simulink model "SF049A_LoaMgr"  (R2013b)
settings: Solver=FixedStepDiscrete  SolverMode=SingleTasking  StartTime=0.0  StopTime=1  FixedStep=0.002  RelTol=1e-3
undefined symbols (not defined in the file): CURRMEASLOAMTGTNMASK_CNT_U08, IVTRLOAMTGTNMASK_CNT_U08, LoaCtrldShtdwn, LoaCurrMeasIdptSigNrFlt, LoaHwTqIdptSigNrFlt, LoaImdtShtdwn, LoaIvtrIdptSigNrFlt, LOAMAXSLEW_ULSPERSEC_F32, LoaMgrCurrIvtrMtgtnRate, LoaMgrCurrIvtrMtgtnSca, LoaMgrCurrIvtrMtgtnScaZeroEna, LoaMgrCurrMeasIdptSig0Resp, LoaMgrCurrMeasIdptSig1Resp, LoaMgrCurrMeasIdptSig2Resp, LoaMgrCurrMeasIdptSigFltThd, LoaMgrCurrMeasMtgtnRate, LoaMgrCurrMeasMtgtnSca, LoaMgrCurrMeasMtgtnScaZeroEna, LoaMgrFadeOutStRate, LoaMgrHwTqIdptSig0NoTqLoaResp, LoaMgrHwTqIdptSig1NoTqLoaResp, LoaMgrHwTqIdptSig2Resp, LoaMgrHwTqIdptSig4Resp, LoaMgrHwTqIdptSigFltThd, LoaMgrHwTqLoaAvlResp, LoaMgrIvtrIdptSig0Resp, LoaMgrIvtrIdptSig1Resp, LoaMgrIvtrIdptSig2Resp, LoaMgrIvtrIdptSigFltThd, LoaMgrIvtrMtgtnRate, LoaMgrIvtrMtgtnSca, LoaMgrIvtrMtgtnScaZeroEna, LoaMgrLimdStRate, LoaMgrLimdStSca, LoaMgrMotAgAvlSnsrlsResp, LoaMgrMotAgIdptSig0NoSnsrlsResp, LoaMgrMotAgIdptSig1NoSnsrlsResp, LoaMgrMotAgIdptSig2Resp, LoaMgrMotAgIdptSig3Resp, LoaMgrMotAgIdptSigFltThd, LoaMgrMotAgMtgtnRate, LoaMgrMotAgMtgtnSca, LoaMgrMotAgMtgtnScaZeroEna, LoaMotAgIdptSigNrFlt, LOASCAONE_ULS_F32, LOASCAZERO_ULS_F32, LoaSt1, LOASTIMDTSHTDWN_CNT_U08, LOASTNORM_CNT_U08, LOASTSWMTGTN_CNT_U08, MAXCURRMEASIDPTSIGALLWD_CNT_U08, MAXHWTQIDPTSIGALLWD_CNT_U08, MAXIVTRIDPTSIGALLWD_CNT_U08, MAXMOTAGMECLIDPTSIGALLWD_CNT_U08, NODEBSTEP_CNT_U16, NtcSts1, SigQlfr1
libraries: simulink x30, NxtrMin x4, NxtrMax x4, NxtrLim x2
(part 1 of 7)
settings Model: Creator=TZ5743  LastModifiedBy=BZHF94
settings SolverCC: AutoInsertRateTranBlk=on  InsertRTBMode=Always
settings DataIOCC: LimitDataPoints=off  SaveFormat=Structure  ReturnWorkspaceOutputs=on
settings OptimizationCC: BlockReduction=off  DefaultParameterBehavior=Inlined  ZeroExternalMemoryAtStartup=off  ZeroInternalMemoryAtStartup=off  OptimizeModelRefInitCode=on  LifeSpan=1  SimCompilerOptimization=off
settings DebuggingCC: SignalInfNanChecking=error  SignalRangeChecking=warning  UnderspecifiedInitializationDetection=Simplified  MergeDetectMultiDrivingBlocksExec=error  SolverPrmCheckMsg=error  InheritedTsInSrcMsg=error  SingleTaskRateTransMsg=error  TasksWithSamePriorityMsg=error  SigSpecEnsureSampleTimeMsg=error  CheckMatrixSingularityMsg=error  ParameterUnderflowMsg=error  ParameterPrecisionLossMsg=error  ParameterTunabilityLossMsg=error  FixptConstUnderflowMsg=warning  FixptConstOverflowMsg=warning  VectorMatrixConversionMsg=error  SignalLabelMismatchMsg=error  UnconnectedInputMsg=error  UnconnectedOutputMsg=error  UnconnectedLineMsg=error  SFcnCompatibilityMsg=error  FrameProcessingCompatibilityMsg=error  UniqueDataStoreMsg=warning  BusObjectLabelMismatch=error  RootOutportRequireBusObject=error  AssertControl=DisableAll  AllowSymbolicDim=off  ModelReferenceIOMsg=error  ModelReferenceVersionMismatchMessage=warning  ModelReferenceIOMismatchMessage=error  ModelReferenceDataLoggingMessage=error  StateNameClashWarn=warning  StrictBusMsg=ErrorOnBusTreatedAsVector  NonBusSignalsTreatedAsBus=error  SFUnexpectedBacktrackingDiag=error  SFInvalidInputDataAccessInChartInitDiag=error  SFNoUnconditionalDefaultTransitionDiag=error  SFTransitionOutsideNaturalParentDiag=error  SFUnconditionalTransitionShadowingDiag=error  SFUndirectedBroadcastEventsDiag=error
settings ModelReferenceCC: ModelReferenceNumInstancesAllowed=Single
settings RTWCC: SystemTargetFile=autosar.tlc  GenCodeOnly=on  TemplateMakefile=ert_default_tmf  Description=AUTOSAR  GenerateReport=on  LaunchReport=on  RTWCompilerOptimization=off
settings CodeAppCC: GenerateComments=off  IgnoreCustomStorageClasses=off  CustomSymbolStrType=$N$R$M  CustomSymbolStrBlkIO=$N$M  SimulinkBlockComments=off
settings STFCustomTargetCC: CodeReplacementLibrary=None  ParMdlRefBuildCompliant=on  CompOptLevelCompliant=on  IncludeMdlTerminateFcn=off  CombineOutputUpdateFcns=on  SuppressErrorStatus=on  ERTFirstTimeCompliant=on  ERTCustomFileBanners=on  SupportNonFinite=off  SupportComplex=off  SupportContinuousTime=off  SupportNonInlinedSFcns=off  MATLABClassNameForMDSCustomization=Simulink.SoftwareTarget.ERTCustomization  AutosarCompliant=on  GRTInterface=off  UseToolchainInfoCompliant=on  SystemTargetFile=autosar.tlc
settings ERTTargetCC: ConcurrentExecutionCompliant=off  IncludeMdlTerminateFcn=off  SuppressErrorStatus=on  SupportNonFinite=off  SupportComplex=off  ModelStepFunctionPrototypeControlCompliant=off  CPPClassGenCompliant=off  AutosarCompliant=on  InlinedParameterPlacement=NonHierarchical  ERTCustomFileTemplate=example_file_process.tlc  EnableUserReplacementTypes=on
settings ConfigComp: CovMetricSettings=dw  CovHtmlReporting=on  CovSaveCumulativeToWorkspaceVar=on  CovSaveSingleToWorkspaceVar=on  CovModelRefEnable=Off  CovExternalEMLEnable=off

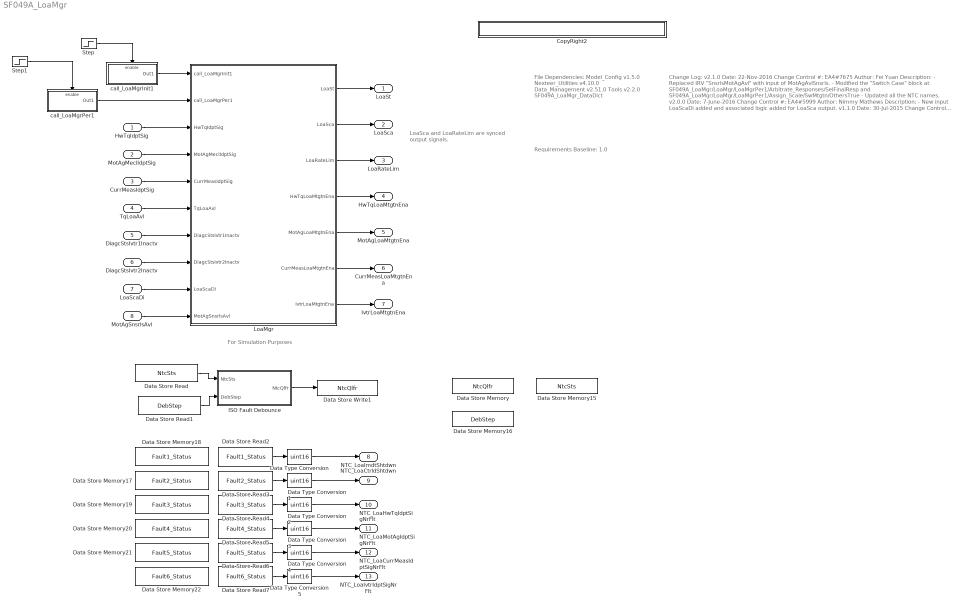
== system SF049A_LoaMgr ==
  note: LoaSca and LoaRateLim are synced
      | output signals.
  note: File Dependencies:
      |
      | Model_Config v1.5.0
      | Nexteer_Utilities v4.10.0
      | Data_Management v2.51.0
      | Tools v2.2.0
      | SF049A_LoaMgr_DataDict
  note: Requirements Baseline: 1.0
  note: Change Log:
      |
      | v2.1.0
      | Date: 22-Nov-2016
      | Change Control #: EA4#7675
      | Author: Fei Yuan
      | Description:
      | - Replaced IRV "SnsrlsMotAgAvl" with input of MotAgAvlSnsrls.
      | - Modified the "Switch Case" block at
      | SF049A_LoaMgr/LoaMgr/LoaMgrPer1/Arbitrate_Responses/SelFinalResp and
      | SF049A_LoaMgr/LoaMgr/LoaMgrPer1/Assign_Scale/SwMtgtn/OthersTrue
      | - Updated all the NTC names.
      |
      | v2.0.0
      | Date: 7-June-2016
      | Change Control #: 	EA4#5999
      | Author:  Nimmy Mathews
      | Description:
      | - New input LoaScaDi added and associated logic added for
      | LoaSca output.
      |
      | v1.1.0
      | Date: 30-Jul-2015
      | Change Control #: EA4#947
      | DRW:  Sudeep Shankar
      | Description:
      | - Initial Release based off of EA3 Version v1.1.0
      | - Output Signal name correction
  note: For Simulation Purposes
  HwTqIdptSig : Inport  RequirementInfo={} %GIDa_c0ada7cc_2a84_41fc_944b_6b17ef65ea9c
  MotAgMeclIdptSig : Inport  RequirementInfo={} %GIDa_73372f4d_c568_47db_aad1_8b4638be1747  Port=2
  CurrMeasIdptSig : Inport  RequirementInfo={} %GIDa_84af9224_d287_43ff_b284_7e5ed6dfb324  Port=3
  TqLoaAvl : Inport  RequirementInfo={} %GIDa_93076217_93fd_4cef_a21d_6480a5a63a27  Port=4
  DiagcStsIvtr1Inactv : Inport  RequirementInfo={} %GIDa_3739eb85_24f0_476e_b882_4900d0ef3f73  Port=5
  DiagcStsIvtr2Inactv : Inport  RequirementInfo={} %GIDa_5f578b66_4982_413b_90dc_34bab3afd1d1  Port=6
  LoaScaDi : Inport  RequirementInfo={} %GIDa_13ee9f09_c993_4f8a_825d_b1ce3d1d2719  Port=7
  MotAgSnsrlsAvl : Inport  RequirementInfo={} %GIDa_1b4fe355_7a68_40b3_bc8e_ac797fbd4766  Port=8
  CopyRight2 : Subsystem  Description=|  mask(Copyright Information){none=on}
      | Copyright info block.                                               
      |                                                                     
      | Place copyright information at the top of every subsystem in design.
      mask prompts: none "No parameters"
      mask help: Place copyright information at the top of every subsystem in design.
      mask Display:
      | NxtrConf = 'Nexteer Confidential';
      | 
      | sys = bdroot; %handle for the current model ("system")
      | first = get_param(sys,'Created');
      | if(isempty(first))
      |     first = datestr(now,'yyyy');
      | else
      |     first = first(end-3:end);  %year is last four digits
      | end
      | 
      | last = get_param(sys,'LastModifiedDate');
      | if isempty(last)
      |     last = datestr(now,'yyyy');
      | else
      |     last = last(end-3:end);
      | end
      | 
      | if strcmp(first,last)
      |     fprintf('%s -- Copyright %s Nexteer',NxtrConf,first)
      | else
      |     fprintf('%s -- %s%s- %s Nexteer',NxtrConf,char(169),first,last)
      | end
  Data Store Memory : DataStoreMemory  DataStoreName=NtcQlfr  OutDataTypeStr=uint8
  Data Store Memory15 : DataStoreMemory  DataStoreName=NtcSts  InitialValue=NtcSts1.NTCSTS_PREPASSD
  Data Store Memory16 : DataStoreMemory  DataStoreName=DebStep
  Data Store Memory17 : DataStoreMemory  DataStoreName=Fault2_Status  InitialValue=NtcSts1.NTCSTS_PASSD  OutDataTypeStr=Enum: NtcSts1
  Data Store Memory18 : DataStoreMemory  DataStoreName=Fault1_Status  InitialValue=NtcSts1.NTCSTS_PASSD  OutDataTypeStr=Enum: NtcSts1
  Data Store Memory19 : DataStoreMemory  DataStoreName=Fault3_Status  InitialValue=NtcSts1.NTCSTS_PASSD  OutDataTypeStr=Enum: NtcSts1
  Data Store Memory20 : DataStoreMemory  DataStoreName=Fault4_Status  InitialValue=NtcSts1.NTCSTS_PASSD  OutDataTypeStr=Enum: NtcSts1
  Data Store Memory21 : DataStoreMemory  DataStoreName=Fault5_Status  InitialValue=NtcSts1.NTCSTS_PASSD  OutDataTypeStr=Enum: NtcSts1
  Data Store Memory22 : DataStoreMemory  DataStoreName=Fault6_Status  InitialValue=NtcSts1.NTCSTS_PASSD  OutDataTypeStr=Enum: NtcSts1
  Data Store Read : DataStoreRead  DataStoreName=NtcSts  SampleTime=0.004
  Data Store Read1 : DataStoreRead  DataStoreName=DebStep  SampleTime=0.004
  Data Store Read2 : DataStoreRead  DataStoreName=Fault1_Status  SampleTime=.004
  Data Store Read3 : DataStoreRead  DataStoreName=Fault2_Status  SampleTime=.004
  Data Store Read4 : DataStoreRead  DataStoreName=Fault3_Status  SampleTime=.004
  Data Store Read5 : DataStoreRead  DataStoreName=Fault4_Status  SampleTime=.004
  Data Store Read6 : DataStoreRead  DataStoreName=Fault5_Status  SampleTime=.004
  Data Store Read7 : DataStoreRead  DataStoreName=Fault6_Status  SampleTime=0.004
  Data Store Write1 : DataStoreWrite  DataStoreName=NtcQlfr
  Data Type Conversion{,1..5} (6 alike) : DataTypeConversion  OutDataTypeStr=uint16
  ISO Fault Debounce : Subsystem  mask(SetNTC){}
      mask help: For Simulation Purposes
  LoaMgr : Subsystem
  Step : Step  Time=.0001  Before=1  After=0  SampleTime=0
  Step1 : Step  Time=.004  SampleTime=0
  call_LoaMgrInit1 : Subsystem  TreatAsAtomicUnit=on
  call_LoaMgrPer1 : Subsystem  TreatAsAtomicUnit=on
  LoaSt : Outport  RequirementInfo={} %GIDa_93bae52a_8cb1_4bd9_a2c4_d588b7d059cf
  LoaSca : Outport  RequirementInfo={} %GIDa_8c460775_12f6_4528_9f51_57ca189e85fc  Port=2
  LoaRateLim : Outport  RequirementInfo={} %GIDa_ffab9872_1ea4_4ffd_9e16_324c719cb008  Port=3
  HwTqLoaMtgtnEna : Outport  RequirementInfo={} %GIDa_b272817b_3ff3_4259_b745_ea4cd35b806a  Port=4
  MotAgLoaMtgtnEna : Outport  RequirementInfo={} %GIDa_98224876_72c1_4d11_a238_725dcb00f091  Port=5
  CurrMeasLoaMtgtnEna : Outport  RequirementInfo={} %GIDa_771c3727_c0e3_4c42_9260_a180eb374e5c  Port=6
  IvtrLoaMtgtnEna : Outport  RequirementInfo={} %GIDa_ccb9de9c_ade8_4e48_bfad_57a91e3cbf19  Port=7
  NTC_LoaImdtShtdwn : Outport  Port=8
  NTC_LoaCtrldShtdwn : Outport  Port=9
  NTC_LoaHwTqIdptSigNrFlt : Outport  Port=10
  NTC_LoaMotAgIdptSigNrFlt : Outport  Port=11
  NTC_LoaCurrMeasIdptSigNrFlt : Outport  Port=12
  NTC_LoaIvtrIdptSigNrFlt : Outport  Port=13
  wires:
  HwTqIdptSig/1 -> LoaMgr/3(HwTqIdptSig)
  MotAgMeclIdptSig/1 -> LoaMgr/4(MotAgMeclIdptSig)
  CurrMeasIdptSig/1 -> LoaMgr/5(CurrMeasIdptSig)
  DiagcStsIvtr1Inactv/1 -> LoaMgr/7(DiagcStsIvtr1Inactv)
  TqLoaAvl/1 -> LoaMgr/6(TqLoaAvl)
  DiagcStsIvtr2Inactv/1 -> LoaMgr/8(DiagcStsIvtr2Inactv)
  LoaMgr/7(IvtrLoaMtgtnEna) -> IvtrLoaMtgtnEna/1
  LoaMgr/6(CurrMeasLoaMtgtnEna) -> CurrMeasLoaMtgtnEna/1
  LoaMgr/5(MotAgLoaMtgtnEna) -> MotAgLoaMtgtnEna/1
  LoaMgr/4(HwTqLoaMtgtnEna) -> HwTqLoaMtgtnEna/1
  LoaMgr/3(LoaRateLim) -> LoaRateLim/1
  LoaMgr/2(LoaSca) -> LoaSca/1
  LoaMgr/1(LoaSt) -> LoaSt/1
  call_LoaMgrInit1/1(Out1) -> LoaMgr/1(call_LoaMgrInit1)
  Step/1 -> call_LoaMgrInit1/Enable
  Data Store Read2/1 -> Data Type Conversion/1
  Data Type Conversion/1 -> NTC_LoaImdtShtdwn/1
  Data Store Read3/1 -> Data Type Conversion1/1
  Data Type Conversion1/1 -> NTC_LoaCtrldShtdwn/1
  Data Store Read4/1 -> Data Type Conversion2/1
  Data Type Conversion2/1 -> NTC_LoaHwTqIdptSigNrFlt/1
  Data Type Conversion3/1 -> NTC_LoaMotAgIdptSigNrFlt/1
  Data Type Conversion4/1 -> NTC_LoaCurrMeasIdptSigNrFlt/1
  Data Store Read5/1 -> Data Type Conversion3/1
  Data Store Read6/1 -> Data Type Conversion4/1
  Data Type Conversion5/1 -> NTC_LoaIvtrIdptSigNrFlt/1
  Data Store Read7/1 -> Data Type Conversion5/1
  ISO Fault Debounce/1(NtcQlfr) -> Data Store Write1/1
  Data Store Read/1 -> ISO Fault Debounce/1(NtcSts)
  Data Store Read1/1 -> ISO Fault Debounce/2(DebStep)
  LoaScaDi/1 -> LoaMgr/9(LoaScaDi)
  MotAgSnsrlsAvl/1 -> LoaMgr/10(MotAgSnsrlsAvl)
  Step1/1 -> call_LoaMgrPer1/Enable
  call_LoaMgrPer1/1(Out1) -> LoaMgr/2(call_LoaMgrPer1)

== system SF049A_LoaMgr/CopyRight2 ==

== system SF049A_LoaMgr/ISO Fault Debounce ==
  note: Note:
      |
      | - "ISO Fault Debounce Design" Simulink block intent to use here for Simulation purpose only. Do not Code this block
  NtcSts : Inport
  DebStep : Inport  Port=2
  Constant : Constant  Value=false
  CopyRight2 : Subsystem  Description=|  mask(Copyright Information){none=on}
      | Copyright info block.                                               
      |                                                                     
      | Place copyright information at the top of every subsystem in design.
      mask prompts: none "No parameters"
      mask help: Place copyright information at the top of every subsystem in design.
      mask Display:
      | NxtrConf = 'Nexteer Confidential';
      | 
      | sys = bdroot; %handle for the current model ("system")
      | first = get_param(sys,'Created');
      | first = first(end-3:end);  %year is last four digits
      | 
      | last = get_param(sys,'LastModifiedDate');
      | if isempty(last)
      |     last = datestr(now,'yyyy');
      | else
      |     last = last(end-3:end);
      | end
      | 
      | if strcmp(first,last)
      |     fprintf('%s -- Copyright %s Nexteer',NxtrConf,first)
      | else
      |     fprintf('%s -- %s%s- %s Nexteer',NxtrConf,char(169),first,last)
      | end
  Data Type Conversion : DataTypeConversion
  DiagMgr : Subsystem  RequirementInfo={} %GIDa_61294fe9_bc00_4ee8_bc9f_a9abb89fc5dc
  Ground : Ground
  Terminator : Terminator
  NtcQlfr : Outport
  wires:
  Ground/1 -> DiagMgr/3(SvcClr)
  DebStep/1 -> DiagMgr/2(DebStep)
  NtcSts/1 -> DiagMgr/1(NtcSts)
  Constant/1 -> DiagMgr/4(Recoverable)
  Data Type Conversion/1 -> NtcQlfr/1
  DiagMgr/1(Qualifier) -> Data Type Conversion/1
  DiagMgr/2(ErrAcc) -> Terminator/1

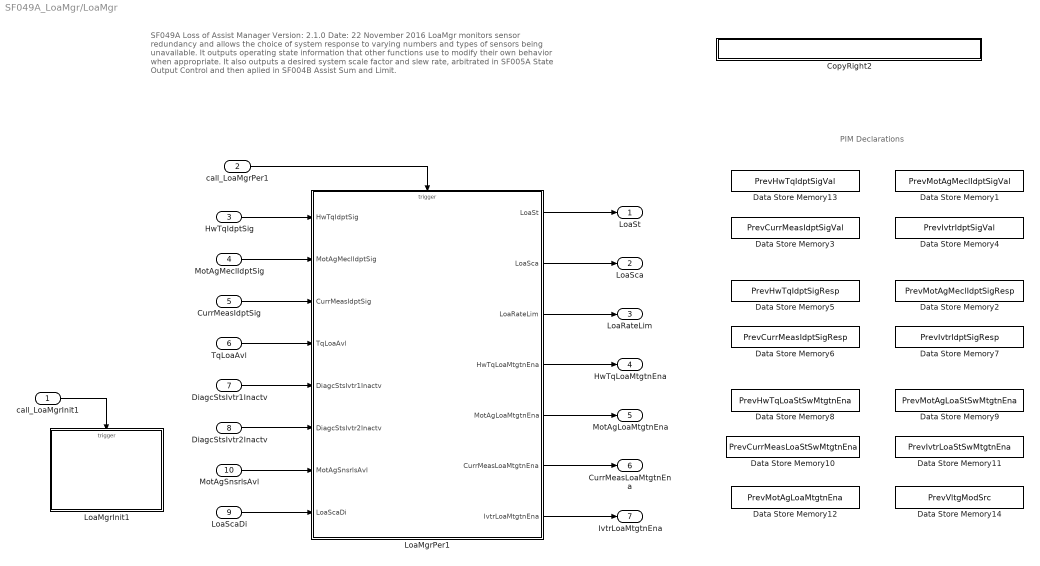
== system SF049A_LoaMgr/LoaMgr ==
  note: SF049A  Loss of Assist Manager       Version: 2.1.0                                                       Date:  22 November 2016
      |
      | LoaMgr monitors sensor redundancy and allows the choice of system response to varying numbers and types of sensors being unavailable.  It
      | outputs operating state information that other functions use to modify their own behavior when appropriate.  It also outputs a desired system
      | scale factor and slew rate, arbitrated in SF005A State Output Control and then aplied in SF004B Assist Sum and Limit.
  note: PIM Declarations
  call_LoaMgrInit1 : Inport
  call_LoaMgrPer1 : Inport  RequirementInfo="{'linktype_rmi_doors' '00012fd5 (/E-STEER Core/SubSystem Specifications/Application Functions - EA4/SF049A Loss of Assist Manager)' '#SF049A_161' 'true' 'REQ:  SF049A_161' '' } %GIDa_11a999fa_4307_4876_8422_1fdf0f90e9d7"  Port=2
  HwTqIdptSig : Inport  RequirementInfo="{'linktype_rmi_doors' '00012fd5 (/E-STEER Core/SubSystem Specifications/Application Functions - EA4/SF049A Loss of Assist Manager)' '#SF049A_9' 'true' 'REQ:  SF049A_9' '' } %GIDa_e136a68a_be9b_41e2_8d19_731d1b546a22"  Port=3
  MotAgMeclIdptSig : Inport  RequirementInfo="{'linktype_rmi_doors' '00012fd5 (/E-STEER Core/SubSystem Specifications/Application Functions - EA4/SF049A Loss of Assist Manager)' '#SF049A_10' 'true' 'REQ:  SF049A_10' '' } %GIDa_03485ada_2d02_4097_843d_27b3dd3d89ce"  Port=4
  CurrMeasIdptSig : Inport  RequirementInfo="{'linktype_rmi_doors' '00012fd5 (/E-STEER Core/SubSystem Specifications/Application Functions - EA4/SF049A Loss of Assist Manager)' '#SF049A_11' 'true' 'REQ:  SF049A_11' '' } %GIDa_b13fb45e_c676_4df0_b1a7_3991e4929c24"  Port=5
  TqLoaAvl : Inport  RequirementInfo="{'linktype_rmi_doors' '00012fd5 (/E-STEER Core/SubSystem Specifications/Application Functions - EA4/SF049A Loss of Assist Manager)' '#SF049A_12' 'true' 'REQ:  SF049A_12' '' } %GIDa_ad428560_d84e_4090_8b2c_395c8b1d79f4"  Port=6
  DiagcStsIvtr1Inactv : Inport  RequirementInfo="{'linktype_rmi_doors' '00012fd5 (/E-STEER Core/SubSystem Specifications/Application Functions - EA4/SF049A Loss of Assist Manager)' '#SF049A_13' 'true' 'REQ:  SF049A_13' '' } %GIDa_a09d3721_2ae3_425a_97fe_a373142e0df8"  Port=7
  DiagcStsIvtr2Inactv : Inport  RequirementInfo="{'linktype_rmi_doors' '00012fd5 (/E-STEER Core/SubSystem Specifications/Application Functions - EA4/SF049A Loss of Assist Manager)' '#SF049A_14' 'true' 'REQ:  SF049A_14' '' } %GIDa_37cf1e87_9470_44c4_ae46_3d3e796de4ab"  Port=8
  LoaScaDi : Inport  RequirementInfo="{'linktype_rmi_doors' '00012fd5 (/E-STEER Core/SubSystem Specifications/Application Functions - EA4/SF049A Loss of Assist Manager)' '#SF049A_15' 'true' 'REQ:  SF049A_15' '' } %GIDa_542c339e_a191_413c_b7b4_dd829497f318"  Port=9
  MotAgSnsrlsAvl : Inport  RequirementInfo="{'linktype_rmi_doors' '00012fd5 (/E-STEER Core/SubSystem Specifications/Application Functions - EA4/SF049A Loss of Assist Manager)' '#SF049A_164' 'true' 'REQ:  SF049A_164' '' } %GIDa_fe7b95aa_5b28_4b7e_a407_a916842b11d1"  Port=10
  CopyRight2 : Subsystem  Description=|  mask(Copyright Information){none=on}
      | Copyright info block.                                               
      |                                                                     
      | Place copyright information at the top of every subsystem in design.
      mask prompts: none "No parameters"
      mask help: Place copyright information at the top of every subsystem in design.
      mask Display:
      | NxtrConf = 'Nexteer Confidential';
      | 
      | sys = bdroot; %handle for the current model ("system")
      | first = get_param(sys,'Created');
      | first = first(end-3:end);  %year is last four digits
      | 
      | last = get_param(sys,'LastModifiedDate');
      | if isempty(last)
      |     last = datestr(now,'yyyy');
      | else
      |     last = last(end-3:end);
      | end
      | 
      | if strcmp(first,last)
      |     fprintf('%s -- Copyright %s Nexteer',NxtrConf,first)
      | else
      |     fprintf('%s -- %s%s- %s Nexteer',NxtrConf,char(169),first,last)
      | end
  Data Store Memory1 : DataStoreMemory  DataStoreName=PrevMotAgMeclIdptSigVal  StateMustResolveToSignalObject=on
  Data Store Memory10 : DataStoreMemory  DataStoreName=PrevCurrMeasLoaStSwMtgtnEna  StateMustResolveToSignalObject=on
  Data Store Memory11 : DataStoreMemory  DataStoreName=PrevIvtrLoaStSwMtgtnEna  StateMustResolveToSignalObject=on
  Data Store Memory12 : DataStoreMemory  DataStoreName=PrevMotAgLoaMtgtnEna  StateMustResolveToSignalObject=on
  Data Store Memory13 : DataStoreMemory  DataStoreName=PrevHwTqIdptSigVal  StateMustResolveToSignalObject=on
  Data Store Memory14 : DataStoreMemory  DataStoreName=PrevVltgModSrc  StateMustResolveToSignalObject=on
  Data Store Memory2 : DataStoreMemory  DataStoreName=PrevMotAgMeclIdptSigResp  StateMustResolveToSignalObject=on
  Data Store Memory3 : DataStoreMemory  DataStoreName=PrevCurrMeasIdptSigVal  StateMustResolveToSignalObject=on
  Data Store Memory4 : DataStoreMemory  DataStoreName=PrevIvtrIdptSigVal  StateMustResolveToSignalObject=on
  Data Store Memory5 : DataStoreMemory  DataStoreName=PrevHwTqIdptSigResp  StateMustResolveToSignalObject=on
  Data Store Memory6 : DataStoreMemory  DataStoreName=PrevCurrMeasIdptSigResp  StateMustResolveToSignalObject=on
  Data Store Memory7 : DataStoreMemory  DataStoreName=PrevIvtrIdptSigResp  StateMustResolveToSignalObject=on
  Data Store Memory8 : DataStoreMemory  DataStoreName=PrevHwTqLoaStSwMtgtnEna  StateMustResolveToSignalObject=on
  Data Store Memory9 : DataStoreMemory  DataStoreName=PrevMotAgLoaStSwMtgtnEna  StateMustResolveToSignalObject=on
  LoaMgrInit1 : Subsystem  TreatAsAtomicUnit=on
  LoaMgrPer1 : Subsystem
  LoaSt : Outport  RequirementInfo="{'linktype_rmi_doors' '00012fd5 (/E-STEER Core/SubSystem Specifications/Application Functions - EA4/SF049A Loss of Assist Manager)' '#SF049A_17' 'true' 'REQ:  SF049A_17' '' } %GIDa_485d87b4_d02d_47fa_b823_48b3336f7452"
  LoaSca : Outport  RequirementInfo="{'linktype_rmi_doors' '00012fd5 (/E-STEER Core/SubSystem Specifications/Application Functions - EA4/SF049A Loss of Assist Manager)' '#SF049A_18' 'true' 'REQ:  SF049A_18' '' } %GIDa_0bd5c46e_7ba7_4668_acb6_e4652e0a23fd"  Port=2
  LoaRateLim : Outport  RequirementInfo="{'linktype_rmi_doors' '00012fd5 (/E-STEER Core/SubSystem Specifications/Application Functions - EA4/SF049A Loss of Assist Manager)' '#SF049A_19' 'true' 'REQ:  SF049A_19' '' } %GIDa_80797401_dd21_4a69_8582_3227909dc8d3"  Port=3
  HwTqLoaMtgtnEna : Outport  RequirementInfo="{'linktype_rmi_doors' '00012fd5 (/E-STEER Core/SubSystem Specifications/Application Functions - EA4/SF049A Loss of Assist Manager)' '#SF049A_20' 'true' 'REQ:  SF049A_20' '' } %GIDa_f23d32ba_f930_49ed_92e7_19e481e9c810"  Port=4
  MotAgLoaMtgtnEna : Outport  RequirementInfo="{'linktype_rmi_doors' '00012fd5 (/E-STEER Core/SubSystem Specifications/Application Functions - EA4/SF049A Loss of Assist Manager)' '#SF049A_21' 'true' 'REQ:  SF049A_21' '' } %GIDa_58615b08_5037_4791_88b8_f139534e2d3d"  Port=5
  CurrMeasLoaMtgtnEna : Outport  RequirementInfo="{'linktype_rmi_doors' '00012fd5 (/E-STEER Core/SubSystem Specifications/Application Functions - EA4/SF049A Loss of Assist Manager)' '#SF049A_22' 'true' 'REQ:  SF049A_22' '' } %GIDa_49e649da_286c_497e_8c32_683faa7a42a6"  Port=6
  IvtrLoaMtgtnEna : Outport  RequirementInfo="{'linktype_rmi_doors' '00012fd5 (/E-STEER Core/SubSystem Specifications/Application Functions - EA4/SF049A Loss of Assist Manager)' '#SF049A_23' 'true' 'REQ:  SF049A_23' '' } %GIDa_de65f1b1_1a81_47b6_87b6_d026873f8ac5"  Port=7
  wires:
  LoaScaDi/1 -> LoaMgrPer1/8(LoaScaDi)
  LoaMgrPer1/1(LoaSt) -> LoaSt/1
  LoaMgrPer1/2(LoaSca) -> LoaSca/1
  LoaMgrPer1/3(LoaRateLim) -> LoaRateLim/1
  LoaMgrPer1/4(HwTqLoaMtgtnEna) -> HwTqLoaMtgtnEna/1
  LoaMgrPer1/5(MotAgLoaMtgtnEna) -> MotAgLoaMtgtnEna/1
  LoaMgrPer1/6(CurrMeasLoaMtgtnEna) -> CurrMeasLoaMtgtnEna/1
  LoaMgrPer1/7(IvtrLoaMtgtnEna) -> IvtrLoaMtgtnEna/1
  call_LoaMgrPer1/1 -> LoaMgrPer1/Trigger
  MotAgMeclIdptSig/1 -> LoaMgrPer1/2(MotAgMeclIdptSig)
  HwTqIdptSig/1 -> LoaMgrPer1/1(HwTqIdptSig)
  TqLoaAvl/1 -> LoaMgrPer1/4(TqLoaAvl)
  DiagcStsIvtr1Inactv/1 -> LoaMgrPer1/5(DiagcStsIvtr1Inactv)
  CurrMeasIdptSig/1 -> LoaMgrPer1/3(CurrMeasIdptSig)
  DiagcStsIvtr2Inactv/1 -> LoaMgrPer1/6(DiagcStsIvtr2Inactv)
  call_LoaMgrInit1/1 -> LoaMgrInit1/Trigger
  MotAgSnsrlsAvl/1 -> LoaMgrPer1/7(MotAgSnsrlsAvl)

== system SF049A_LoaMgr/call_LoaMgrInit1 ==
  Enable : EnablePort
  CopyRight2 : Subsystem  Description=|  mask(Copyright Information){none=on}
      | Copyright info block.                                               
      |                                                                     
      | Place copyright information at the top of every subsystem in design.
      mask prompts: none "No parameters"
      mask help: Place copyright information at the top of every subsystem in design.
      mask Display:
      | NxtrConf = 'Nexteer Confidential';
      | 
      | sys = bdroot; %handle for the current model ("system")
      | first = get_param(sys,'Created');
      | if(isempty(first))
      |     first = datestr(now,'yyyy');
      | else
      |     first = first(end-3:end);  %year is last four digits
      | end
      | 
      | last = get_param(sys,'LastModifiedDate');
      | if isempty(last)
      |     last = datestr(now,'yyyy');
      | else
      |     last = last(end-3:end);
      | end
      | 
      | if strcmp(first,last)
      |     fprintf('%s -- Copyright %s Nexteer',NxtrConf,first)
      | else
      |     fprintf('%s -- %s%s- %s Nexteer',NxtrConf,char(169),first,last)
      | end
  Function-Call Generator : simulink/Ports & Subsystems/Function-Call Generator  sample_time=0  numberOfIterations=1
  Out1 : Outport
  wires:
  Function-Call Generator/1 -> Out1/1

== system SF049A_LoaMgr/call_LoaMgrPer1 ==
  Enable : EnablePort
  CopyRight2 : Subsystem  Description=|  mask(Copyright Information){none=on}
      | Copyright info block.                                               
      |                                                                     
      | Place copyright information at the top of every subsystem in design.
      mask prompts: none "No parameters"
      mask help: Place copyright information at the top of every subsystem in design.
      mask Display:
      | NxtrConf = 'Nexteer Confidential';
      | 
      | sys = bdroot; %handle for the current model ("system")
      | first = get_param(sys,'Created');
      | if(isempty(first))
      |     first = datestr(now,'yyyy');
      | else
      |     first = first(end-3:end);  %year is last four digits
      | end
      | 
      | last = get_param(sys,'LastModifiedDate');
      | if isempty(last)
      |     last = datestr(now,'yyyy');
      | else
      |     last = last(end-3:end);
      | end
      | 
      | if strcmp(first,last)
      |     fprintf('%s -- Copyright %s Nexteer',NxtrConf,first)
      | else
      |     fprintf('%s -- %s%s- %s Nexteer',NxtrConf,char(169),first,last)
      | end
  Function-Call Generator : simulink/Ports & Subsystems/Function-Call Generator  sample_time=0.004  numberOfIterations=1
  Out1 : Outport
  wires:
  Function-Call Generator/1 -> Out1/1

== system SF049A_LoaMgr/ISO Fault Debounce/CopyRight2 ==

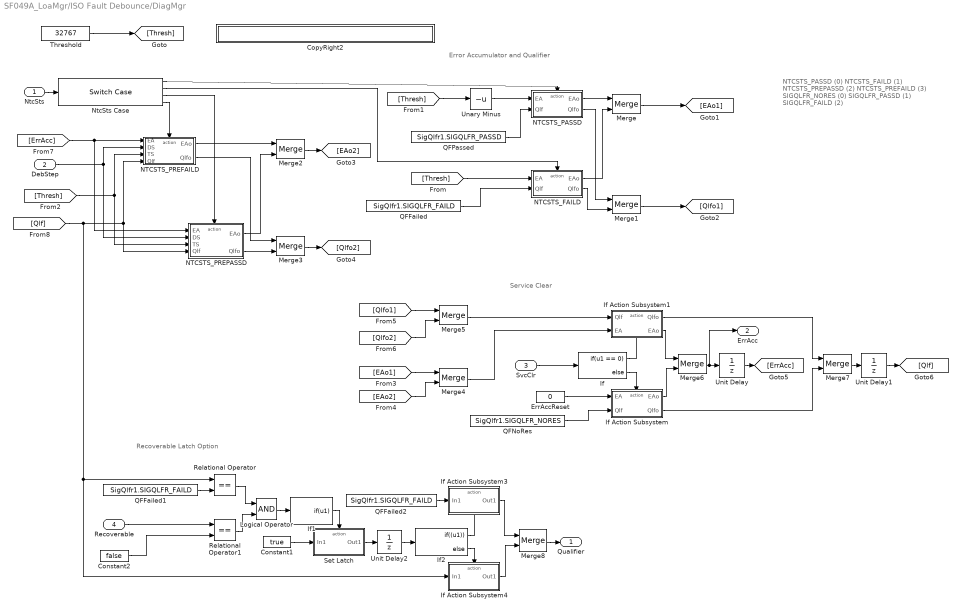
== system SF049A_LoaMgr/ISO Fault Debounce/DiagMgr ==
  note: NTCSTS_PASSD         (0)
      | NTCSTS_FAILD           (1)
      | NTCSTS_PREPASSD  (2)
      | NTCSTS_PREFAILD    (3)
      |
      | SIGQLFR_NORES       (0)
      | SIGQLFR_PASSD        (1)
      | SIGQLFR_FAILD          (2)
  note: Error Accumulator and Qualifier
  note: Service Clear
  note: Recoverable Latch Option
  NtcSts : Inport
  DebStep : Inport  Port=2
  SvcClr : Inport  Port=3
  Recoverable : Inport  Port=4
  Constant1 : Constant  Value=true  OutDataTypeStr=boolean
  Constant2 : Constant  Value=false  OutDataTypeStr=boolean
  CopyRight2 : Subsystem  Description=|  mask(Copyright Information){none=on}
      | Copyright info block.                                               
      |                                                                     
      | Place copyright information at the top of every subsystem in design.
      mask prompts: none "No parameters"
      mask help: Place copyright information at the top of every subsystem in design.
      mask Display:
      | NxtrConf = 'Nexteer Confidential';
      | 
      | sys = bdroot; %handle for the current model ("system")
      | first = get_param(sys,'Created');
      | first = first(end-3:end);  %year is last four digits
      | 
      | last = get_param(sys,'LastModifiedDate');
      | if isempty(last)
      |     last = datestr(now,'yyyy');
      | else
      |     last = last(end-3:end);
      | end
      | 
      | if strcmp(first,last)
      |     fprintf('%s -- Copyright %s Nexteer',NxtrConf,first)
      | else
      |     fprintf('%s -- %s%s- %s Nexteer',NxtrConf,char(169),first,last)
      | end
  ErrAccReset : Constant  Value=0
  If : If  IfExpression=u1 == 0
  If Action Subsystem : Subsystem  TreatAsAtomicUnit=on
  If Action Subsystem1 : Subsystem  TreatAsAtomicUnit=on
  If Action Subsystem3 : Subsystem  TreatAsAtomicUnit=on
  If Action Subsystem4 : Subsystem  TreatAsAtomicUnit=on
  If1 : If  IfExpression=u1  ShowElse=off
  If2 : If  IfExpression=(u1)
  Logical Operator : Logic  AllPortsSameDT=off  OutDataTypeStr=boolean
  Merge{,1..8} (9 alike) : Merge
  NTCSTS_FAILD : Subsystem  TreatAsAtomicUnit=on
  NTCSTS_PASSD : Subsystem  TreatAsAtomicUnit=on
  NTCSTS_PREFAILD : Subsystem  TreatAsAtomicUnit=on
  NTCSTS_PREPASSD : Subsystem  TreatAsAtomicUnit=on
  NtcSts Case : SwitchCase  CaseConditions={NtcSts1.NTCSTS_PASSD,NtcSts1.NTCSTS_FAILD,NtcSts1.NTCSTS_PREPASSD,NtcSts1.NTCSTS_PREFAILD}  ShowDefaultCase=off
  QFFailed : Constant  Value=SigQlfr1.SIGQLFR_FAILD  OutDataTypeStr=Enum: SigQlfr1
  QFFailed1 : Constant  Value=SigQlfr1.SIGQLFR_FAILD  OutDataTypeStr=Enum: SigQlfr1
  QFFailed2 : Constant  Value=SigQlfr1.SIGQLFR_FAILD  OutDataTypeStr=Enum: SigQlfr1
  QFNoRes : Constant  Value=SigQlfr1.SIGQLFR_NORES  OutDataTypeStr=Enum: SigQlfr1
  QFPassed : Constant  Value=SigQlfr1.SIGQLFR_PASSD  OutDataTypeStr=Enum: SigQlfr1
  Relational Operator : RelationalOperator  Operator===  OutDataTypeStr=boolean
      settings: AttributesFormatString=Qualifier Failed
  Relational Operator1 : RelationalOperator  Operator===  OutDataTypeStr=boolean
      settings: AttributesFormatString=Recoverable False
  Set Latch : Subsystem  TreatAsAtomicUnit=on
  Threshold : Constant  Value=32767
  Unary Minus : UnaryMinus
  Unit Delay : UnitDelay  SampleTime=-1
  Unit Delay1 : UnitDelay  InitialCondition=SigQlfr1.SIGQLFR_NORES  SampleTime=-1  StateName=SigQlfr1
  Unit Delay2 : UnitDelay  SampleTime=-1
  Qualifier : Outport
  ErrAcc : Outport  Port=2
  wires:
  DebStep/1 -> NTCSTS_PREPASSD/2(DS), NTCSTS_PREFAILD/2(DS)
  NtcSts Case/3 -> NTCSTS_PREPASSD/Action
  If/2 -> If Action Subsystem/Action
  QFPassed/1 -> NTCSTS_PASSD/2(Qlf)
  If2/1 -> If Action Subsystem3/Action
  If2/2 -> If Action Subsystem4/Action
  [Thresh] -> NTCSTS_FAILD/1(EA)
  QFFailed/1 -> NTCSTS_FAILD/2(Qlf)
  If Action Subsystem4/1(Out1) -> Merge8/2
  Merge8/1 -> Qualifier/1
  QFFailed2/1 -> If Action Subsystem3/1(In1)
  Unit Delay2/1 -> If2/1
  NtcSts Case/1 -> NTCSTS_PASSD/Action
  NtcSts Case/4 -> NTCSTS_PREFAILD/Action
  SvcClr/1 -> If/1
  NtcSts Case/2 -> NTCSTS_FAILD/Action
  [Thresh] -> Unary Minus/1
  [Thresh] -> NTCSTS_PREPASSD/3(TS), NTCSTS_PREFAILD/3(TS)
  NTCSTS_PREFAILD/2(Qlfo) -> Merge3/1
  [ErrAcc] -> NTCSTS_PREPASSD/1(EA), NTCSTS_PREFAILD/1(EA)
  NTCSTS_PREPASSD/1(EAo) -> Merge2/2
  NTCSTS_FAILD/1(EAo) -> Merge/2
  NTCSTS_FAILD/2(Qlfo) -> Merge1/2
  If Action Subsystem3/1(Out1) -> Merge8/1
  [Qlfo1] -> Merge5/1
  NTCSTS_PREPASSD/2(Qlfo) -> Merge3/2
  NTCSTS_PREFAILD/1(EAo) -> Merge2/1
  [Qlfo2] -> Merge5/2
  [EAo1] -> Merge4/1
  [Qlf] -> Relational Operator/1, If Action Subsystem4/1(In1), NTCSTS_PREFAILD/4(Qlf), NTCSTS_PREPASSD/4(Qlf)
  [EAo2] -> Merge4/2
  Merge/1 -> [EAo1]
  ErrAccReset/1 -> If Action Subsystem/1(EA)
  QFNoRes/1 -> If Action Subsystem/2(Qlf)
  Merge6/1 -> ErrAcc/1, Unit Delay/1
  If Action Subsystem1/2(EAo) -> Merge6/1
  Merge4/1 -> If Action Subsystem1/2(EA)
  If/1 -> If Action Subsystem1/Action
  If Action Subsystem1/1(Qlfo) -> Merge7/1
  NTCSTS_PASSD/2(Qlfo) -> Merge1/1
  Threshold/1 -> [Thresh]
  If Action Subsystem/1(EAo) -> Merge6/2
  NTCSTS_PASSD/1(EAo) -> Merge/1
  If Action Subsystem/2(Qlfo) -> Merge7/2
  Merge1/1 -> [Qlfo1]
  Merge2/1 -> [EAo2]
  Merge3/1 -> [Qlfo2]
  Merge5/1 -> If Action Subsystem1/1(Qlf)
  NtcSts/1 -> NtcSts Case/1
  Unit Delay/1 -> [ErrAcc]
  Unit Delay1/1 -> [Qlf]
  Merge7/1 -> Unit Delay1/1
  Relational Operator/1 -> Logical Operator/1
  Relational Operator1/1 -> Logical Operator/2
  Constant2/1 -> Relational Operator1/2
  Logical Operator/1 -> If1/1
  If1/1 -> Set Latch/Action
  Constant1/1 -> Set Latch/1(In1)
  QFFailed1/1 -> Relational Operator/2
  Set Latch/1(Out1) -> Unit Delay2/1
  Recoverable/1 -> Relational Operator1/1
  Unary Minus/1 -> NTCSTS_PASSD/1(EA)

== system SF049A_LoaMgr/LoaMgr/CopyRight2 ==

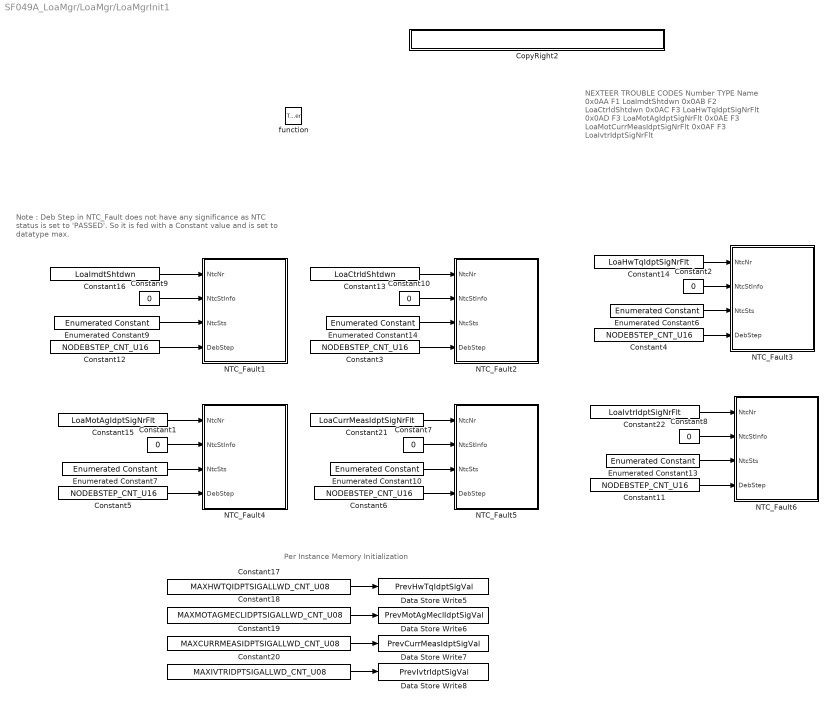
== system SF049A_LoaMgr/LoaMgr/LoaMgrInit1 ==
  note: Per Instance Memory Initialization
  note: NEXTEER TROUBLE CODES
      | Number  TYPE   Name
      |  0x0AA      F1      LoaImdtShtdwn
      |  0x0AB      F2      LoaCtrldShtdwn
      |  0x0AC      F3      LoaHwTqIdptSigNrFlt
      |  0x0AD      F3      LoaMotAgIdptSigNrFlt
      |  0x0AE      F3      LoaMotCurrMeasIdptSigNrFlt
      |  0x0AF      F3      LoaIvtrIdptSigNrFlt
  note: Note : Deb Step in NTC_Fault does not have any significance as
      | NTC status is set to 'PASSED'. So it is fed with a Constant value and
      | is set to datatype max.
  function : TriggerPort  TriggerType=function-call
  Constant1 : Constant  RequirementInfo="{'linktype_rmi_doors' '00012fd5 (/E-STEER Core/SubSystem Specifications/Application Functions - EA4/SF049A Loss of Assist Manager)' '#SF049A_68' 'true' 'REQ:  SF049A_68' '' } %GIDa_09a72554_6b8b_4627_b610_7c880b96c152"  Value=0
  Constant10 : Constant  RequirementInfo="{'linktype_rmi_doors' '00012fd5 (/E-STEER Core/SubSystem Specifications/Application Functions - EA4/SF049A Loss of Assist Manager)' '#SF049A_46' 'true' 'REQ:  SF049A_46' '' } %GIDa_2780d869_b7d4_4c52_8148_a5ebd8a8c128"  Value=0
  Constant11 : Constant  RequirementInfo="{'linktype_rmi_doors' '00012fd5 (/E-STEER Core/SubSystem Specifications/Application Functions - EA4/SF049A Loss of Assist Manager)' '#SF049A_90' 'true' 'REQ:  SF049A_90' '' } %GIDa_8760c850_a166_4f26_aeef_3d69371a50e7"  Value=NODEBSTEP_CNT_U16
  Constant12 : Constant  RequirementInfo="{'linktype_rmi_doors' '00012fd5 (/E-STEER Core/SubSystem Specifications/Application Functions - EA4/SF049A Loss of Assist Manager)' '#SF049A_35' 'true' 'REQ:  SF049A_35' '' } %GIDa_d176be49_c6f2_4e13_b18e_1b05a48376bf"  Value=NODEBSTEP_CNT_U16
  Constant13 : Constant  RequirementInfo="{'linktype_rmi_doors' '00012fd5 (/E-STEER Core/SubSystem Specifications/Application Functions - EA4/SF049A Loss of Assist Manager)' '#SF049A_46' 'true' 'REQ:  SF049A_46' '' } %GIDa_6c547535_063b_445c_af94_eb5574f08747"  Value=LoaCtrldShtdwn
  Constant14 : Constant  RequirementInfo="{'linktype_rmi_doors' '00012fd5 (/E-STEER Core/SubSystem Specifications/Application Functions - EA4/SF049A Loss of Assist Manager)' '#SF049A_57' 'true' 'REQ:  SF049A_57' '' } %GIDa_6c0d8de0_c077_4a89_b170_495f4d0daf45"  Value=LoaHwTqIdptSigNrFlt
  Constant15 : Constant  RequirementInfo="{'linktype_rmi_doors' '00012fd5 (/E-STEER Core/SubSystem Specifications/Application Functions - EA4/SF049A Loss of Assist Manager)' '#SF049A_68' 'true' 'REQ:  SF049A_68' '' } %GIDa_f4e97660_4a45_4ee8_aefd_216a590e907f"  Value=LoaMotAgIdptSigNrFlt
  Constant16 : Constant  RequirementInfo="{'linktype_rmi_doors' '00012fd5 (/E-STEER Core/SubSystem Specifications/Application Functions - EA4/SF049A Loss of Assist Manager)' '#SF049A_35' 'true' 'REQ:  SF049A_35' '' } %GIDa_ee2f095f_e9fa_486e_ae86_a30232b53fb4"  Value=LoaImdtShtdwn
  Constant17 : Constant  RequirementInfo={} %GIDa_5b950255_8f18_4912_81dd_eb91606197df  Value=MAXHWTQIDPTSIGALLWD_CNT_U08  OutDataTypeStr=uint8
  Constant18 : Constant  RequirementInfo={} %GIDa_54c005ab_4540_429a_9970_f23d45e39613  Value=MAXMOTAGMECLIDPTSIGALLWD_CNT_U08  OutDataTypeStr=uint8
  Constant19 : Constant  RequirementInfo={} %GIDa_947a6b5f_12de_441e_bcec_6b3f89217e6d  Value=MAXCURRMEASIDPTSIGALLWD_CNT_U08  OutDataTypeStr=uint8
  Constant2 : Constant  RequirementInfo="{'linktype_rmi_doors' '00012fd5 (/E-STEER Core/SubSystem Specifications/Application Functions - EA4/SF049A Loss of Assist Manager)' '#SF049A_57' 'true' 'REQ:  SF049A_57' '' } %GIDa_83264d8f_e7cf_4e36_a77c_cbe9ece48f33"  Value=0
  Constant20 : Constant  RequirementInfo={} %GIDa_07837d8e_9d24_42c2_b79b_cfda2d14c87d  Value=MAXIVTRIDPTSIGALLWD_CNT_U08  OutDataTypeStr=uint8
  Constant21 : Constant  RequirementInfo="{'linktype_rmi_doors' '00012fd5 (/E-STEER Core/SubSystem Specifications/Application Functions - EA4/SF049A Loss of Assist Manager)' '#SF049A_79' 'true' 'REQ:  SF049A_79' '' } %GIDa_0ddbf860_f1d0_48af_9661_f573615d1661"  Value=LoaCurrMeasIdptSigNrFlt
  Constant22 : Constant  RequirementInfo="{'linktype_rmi_doors' '00012fd5 (/E-STEER Core/SubSystem Specifications/Application Functions - EA4/SF049A Loss of Assist Manager)' '#SF049A_90' 'true' 'REQ:  SF049A_90' '' } %GIDa_9c0928f8_bb13_48cc_a72b_c39958c4c501"  Value=LoaIvtrIdptSigNrFlt
  Constant3 : Constant  RequirementInfo="{'linktype_rmi_doors' '00012fd5 (/E-STEER Core/SubSystem Specifications/Application Functions - EA4/SF049A Loss of Assist Manager)' '#SF049A_46' 'true' 'REQ:  SF049A_46' '' } %GIDa_0bf69534_0956_44cc_9c2a_433bc6c27e43"  Value=NODEBSTEP_CNT_U16
  Constant4 : Constant  RequirementInfo="{'linktype_rmi_doors' '00012fd5 (/E-STEER Core/SubSystem Specifications/Application Functions - EA4/SF049A Loss of Assist Manager)' '#SF049A_57' 'true' 'REQ:  SF049A_57' '' } %GIDa_0fa24ea6_9c16_40ba_9b81_9df4de3ddc47"  Value=NODEBSTEP_CNT_U16
  Constant5 : Constant  RequirementInfo="{'linktype_rmi_doors' '00012fd5 (/E-STEER Core/SubSystem Specifications/Application Functions - EA4/SF049A Loss of Assist Manager)' '#SF049A_68' 'true' 'REQ:  SF049A_68' '' } %GIDa_29c9f302_3383_4bbb_86ad_bd7246db1c6a"  Value=NODEBSTEP_CNT_U16
  Constant6 : Constant  RequirementInfo="{'linktype_rmi_doors' '00012fd5 (/E-STEER Core/SubSystem Specifications/Application Functions - EA4/SF049A Loss of Assist Manager)' '#SF049A_79' 'true' 'REQ:  SF049A_79' '' } %GIDa_693eee1d_940e_4510_b6ca_b2e09a33882e"  Value=NODEBSTEP_CNT_U16
  Constant7 : Constant  RequirementInfo="{'linktype_rmi_doors' '00012fd5 (/E-STEER Core/SubSystem Specifications/Application Functions - EA4/SF049A Loss of Assist Manager)' '#SF049A_79' 'true' 'REQ:  SF049A_79' '' } %GIDa_bd597d58_e2c2_4d46_a831_7ad8a2d0c9f8"  Value=0
  Constant8 : Constant  RequirementInfo="{'linktype_rmi_doors' '00012fd5 (/E-STEER Core/SubSystem Specifications/Application Functions - EA4/SF049A Loss of Assist Manager)' '#SF049A_90' 'true' 'REQ:  SF049A_90' '' } %GIDa_66b775bc_b9d9_40ba_b454_434fd06622b7"  Value=0
  Constant9 : Constant  RequirementInfo="{'linktype_rmi_doors' '00012fd5 (/E-STEER Core/SubSystem Specifications/Application Functions - EA4/SF049A Loss of Assist Manager)' '#SF049A_35' 'true' 'REQ:  SF049A_35' '' } %GIDa_7a457627_e162_4cd9_b6f0_06929f77b0ee"  Value=0
  CopyRight2 : Subsystem  Description=|  mask(Copyright Information){none=on}
      | Copyright info block.                                               
      |                                                                     
      | Place copyright information at the top of every subsystem in design.
      mask prompts: none "No parameters"
      mask help: Place copyright information at the top of every subsystem in design.
      mask Display:
      | NxtrConf = 'Nexteer Confidential';
      | 
      | sys = bdroot; %handle for the current model ("system")
      | first = get_param(sys,'Created');
      | first = first(end-3:end);  %year is last four digits
      | 
      | last = get_param(sys,'LastModifiedDate');
      | if isempty(last)
      |     last = datestr(now,'yyyy');
      | else
      |     last = last(end-3:end);
      | end
      | 
      | if strcmp(first,last)
      |     fprintf('%s -- Copyright %s Nexteer',NxtrConf,first)
      | else
      |     fprintf('%s -- %s%s- %s Nexteer',NxtrConf,char(169),first,last)
      | end
  Data Store Write5 : DataStoreWrite  RequirementInfo={} %GIDa_6608b05c_0683_4793_b206_c046e47d2e17  DataStoreName=PrevHwTqIdptSigVal
  Data Store Write6 : DataStoreWrite  RequirementInfo={} %GIDa_7f471370_469d_423d_8316_5f647dac324c  DataStoreName=PrevMotAgMeclIdptSigVal
  Data Store Write7 : DataStoreWrite  RequirementInfo={} %GIDa_ff2dc782_9d50_4d1d_a106_f1a00891ebf8  DataStoreName=PrevCurrMeasIdptSigVal
  Data Store Write8 : DataStoreWrite  RequirementInfo={} %GIDa_82eaf6ef_b4dd_4627_9b7c_307f23025eff  DataStoreName=PrevIvtrIdptSigVal
  Enumerated Constant10 : simulink/Sources/Enumerated Constant  RequirementInfo="{'linktype_rmi_doors' '00012fd5 (/E-STEER Core/SubSystem Specifications/Application Functions - EA4/SF049A Loss of Assist Manager)' '#SF049A_79' 'true' 'REQ:  SF049A_79' '' } %GIDa_b526159a_7605_418a_8f6c_df09f8ab0f2e"  OutDataTypeStr=Enum: NtcSts1  Value=NtcSts1.NTCSTS_PASSD  SampleTime=inf
  Enumerated Constant13 : simulink/Sources/Enumerated Constant  RequirementInfo="{'linktype_rmi_doors' '00012fd5 (/E-STEER Core/SubSystem Specifications/Application Functions - EA4/SF049A Loss of Assist Manager)' '#SF049A_90' 'true' 'REQ:  SF049A_90' '' } %GIDa_d3e6efb1_efb4_427f_b5b5_516029acb430"  OutDataTypeStr=Enum: NtcSts1  Value=NtcSts1.NTCSTS_PASSD  SampleTime=inf
  Enumerated Constant14 : simulink/Sources/Enumerated Constant  RequirementInfo="{'linktype_rmi_doors' '00012fd5 (/E-STEER Core/SubSystem Specifications/Application Functions - EA4/SF049A Loss of Assist Manager)' '#SF049A_46' 'true' 'REQ:  SF049A_46' '' } %GIDa_c0c65592_9d54_46fb_86ce_f75ee339a4f0"  OutDataTypeStr=Enum: NtcSts1  Value=NtcSts1.NTCSTS_PASSD  SampleTime=inf
  Enumerated Constant6 : simulink/Sources/Enumerated Constant  RequirementInfo="{'linktype_rmi_doors' '00012fd5 (/E-STEER Core/SubSystem Specifications/Application Functions - EA4/SF049A Loss of Assist Manager)' '#SF049A_57' 'true' 'REQ:  SF049A_57' '' } %GIDa_35a763d2_042b_4007_a721_954fca523208"  OutDataTypeStr=Enum: NtcSts1  Value=NtcSts1.NTCSTS_PASSD  SampleTime=inf
  Enumerated Constant7 : simulink/Sources/Enumerated Constant  RequirementInfo="{'linktype_rmi_doors' '00012fd5 (/E-STEER Core/SubSystem Specifications/Application Functions - EA4/SF049A Loss of Assist Manager)' '#SF049A_68' 'true' 'REQ:  SF049A_68' '' } %GIDa_351ce1e7_b97b_403a_a411_28e1e89dcaf0"  OutDataTypeStr=Enum: NtcSts1  Value=NtcSts1.NTCSTS_PASSD  SampleTime=inf
  Enumerated Constant9 : simulink/Sources/Enumerated Constant  RequirementInfo="{'linktype_rmi_doors' '00012fd5 (/E-STEER Core/SubSystem Specifications/Application Functions - EA4/SF049A Loss of Assist Manager)' '#SF049A_35' 'true' 'REQ:  SF049A_35' '' } %GIDa_30de0318_7c37_4833_8d7b_7440b72a791d"  OutDataTypeStr=Enum: NtcSts1  Value=NtcSts1.NTCSTS_PASSD  SampleTime=inf
  NTC_Fault1 : Subsystem  RequirementInfo="{'linktype_rmi_doors' '00012fd5 (/E-STEER Core/SubSystem Specifications/Application Functions - EA4/SF049A Loss of Assist Manager)' '#SF049A_35' 'true' 'REQ:  SF049A_35' '' } %GIDa_a11aadfb_dddf_46de_834c_f65b067005f1"  mask(SetNTC){}
      mask help: SetNTC library block
  NTC_Fault2 : Subsystem  RequirementInfo="{'linktype_rmi_doors' '00012fd5 (/E-STEER Core/SubSystem Specifications/Application Functions - EA4/SF049A Loss of Assist Manager)' '#SF049A_46' 'true' 'REQ:  SF049A_46' '' } %GIDa_297ee9a4_b750_4631_af05_5b9d8d57969c"  mask(SetNTC){}
      mask help: SetNTC library block
  NTC_Fault3 : Subsystem  RequirementInfo="{'linktype_rmi_doors' '00012fd5 (/E-STEER Core/SubSystem Specifications/Application Functions - EA4/SF049A Loss of Assist Manager)' '#SF049A_57' 'true' 'REQ:  SF049A_57' '' } %GIDa_1a5739c7_318f_4ab5_8a5c_73d329586bde"  mask(SetNTC){}
      mask help: SetNTC library block
  NTC_Fault4 : Subsystem  RequirementInfo="{'linktype_rmi_doors' '00012fd5 (/E-STEER Core/SubSystem Specifications/Application Functions - EA4/SF049A Loss of Assist Manager)' '#SF049A_68' 'true' 'REQ:  SF049A_68' '' } %GIDa_1b246348_21bd_45ae_852b_8bbdfb8cae08"  mask(SetNTC){}
      mask help: SetNTC library block
  NTC_Fault5 : Subsystem  RequirementInfo="{'linktype_rmi_doors' '00012fd5 (/E-STEER Core/SubSystem Specifications/Application Functions - EA4/SF049A Loss of Assist Manager)' '#SF049A_79' 'true' 'REQ:  SF049A_79' '' } %GIDa_796fa8cf_8bbd_45c3_b0fb_56c3c4bb3441"  mask(SetNTC){}
      mask help: SetNTC library block
  NTC_Fault6 : Subsystem  RequirementInfo="{'linktype_rmi_doors' '00012fd5 (/E-STEER Core/SubSystem Specifications/Application Functions - EA4/SF049A Loss of Assist Manager)' '#SF049A_90' 'true' 'REQ:  SF049A_90' '' } %GIDa_a3e32d5c_31c5_476e_951c_0fe301f50025"  mask(SetNTC){}
      mask help: SetNTC library block
  wires:
  Constant3/1 -> NTC_Fault2/4(DebStep)
  Enumerated Constant14/1 -> NTC_Fault2/3(NtcSts)
  Constant13/1 -> NTC_Fault2/1(NtcNr)
  Constant10/1 -> NTC_Fault2/2(NtcStInfo)
  Constant12/1 -> NTC_Fault1/4(DebStep)
  Enumerated Constant9/1 -> NTC_Fault1/3(NtcSts)
  Constant9/1 -> NTC_Fault1/2(NtcStInfo)
  Constant16/1 -> NTC_Fault1/1(NtcNr)
  Constant11/1 -> NTC_Fault6/4(DebStep)
  Enumerated Constant13/1 -> NTC_Fault6/3(NtcSts)
  Constant8/1 -> NTC_Fault6/2(NtcStInfo)
  Constant22/1 -> NTC_Fault6/1(NtcNr)
  Constant6/1 -> NTC_Fault5/4(DebStep)
  Enumerated Constant10/1 -> NTC_Fault5/3(NtcSts)
  Constant7/1 -> NTC_Fault5/2(NtcStInfo)
  Constant21/1 -> NTC_Fault5/1(NtcNr)
  Constant5/1 -> NTC_Fault4/4(DebStep)
  Enumerated Constant7/1 -> NTC_Fault4/3(NtcSts)
  Constant1/1 -> NTC_Fault4/2(NtcStInfo)
  Constant15/1 -> NTC_Fault4/1(NtcNr)
  Constant4/1 -> NTC_Fault3/4(DebStep)
  Enumerated Constant6/1 -> NTC_Fault3/3(NtcSts)
  Constant2/1 -> NTC_Fault3/2(NtcStInfo)
  Constant14/1 -> NTC_Fault3/1(NtcNr)
  Constant20/1 -> Data Store Write8/1
  Constant19/1 -> Data Store Write7/1
  Constant18/1 -> Data Store Write6/1
  Constant17/1 -> Data Store Write5/1

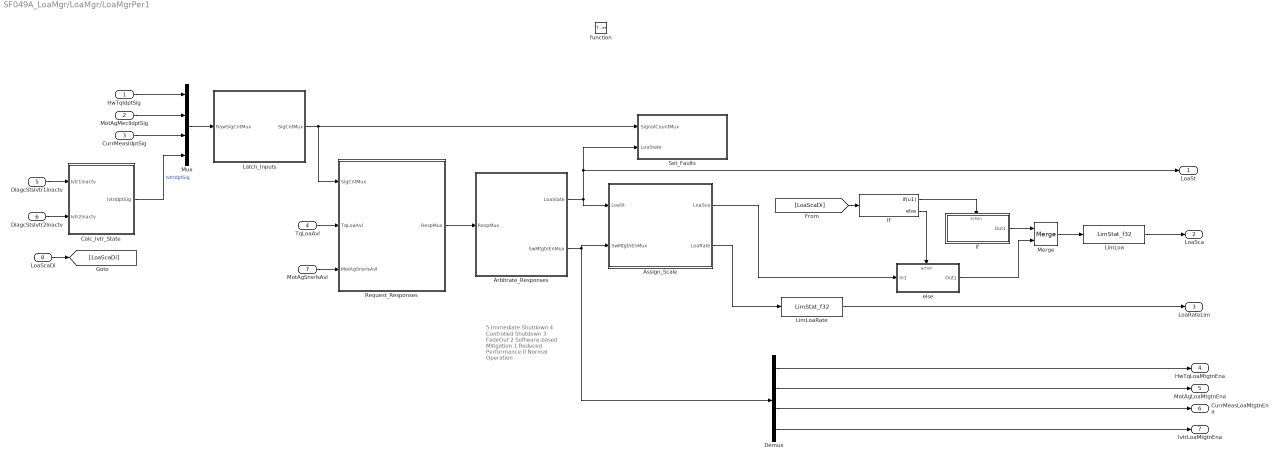
== system SF049A_LoaMgr/LoaMgr/LoaMgrPer1 ==
  note: 5 Immediate Shutdown
      | 4 Controlled Shutdown
      | 3 FadeOut
      | 2 Software-based Mitigation
      | 1 Reduced Performance
      | 0 Normal Operation
  HwTqIdptSig : Inport  RequirementInfo={} %GIDa_5b22ebd4_eebf_4e23_be72_5cf961a78ecc
  MotAgMeclIdptSig : Inport  RequirementInfo={} %GIDa_99431cf8_e55f_4169_aebb_8806cd989f5f  Port=2
  CurrMeasIdptSig : Inport  RequirementInfo={} %GIDa_9762f9cf_e858_4fe8_b88c_9f57261165e8  Port=3
  TqLoaAvl : Inport  RequirementInfo={} %GIDa_7dc665e2_a71f_4a0c_a8d7_522f5f9d9da6  Port=4
  DiagcStsIvtr1Inactv : Inport  RequirementInfo={} %GIDa_1ea8d335_7344_4236_93db_6e2a732118f4  Port=5
  DiagcStsIvtr2Inactv : Inport  RequirementInfo={} %GIDa_ecd8fa16_4ce2_4bf5_a28a_4be529c83f2e  Port=6
  MotAgSnsrlsAvl : Inport  RequirementInfo={} %GIDa_64b909c7_a412_489c_b18f_33829bc3b978  Port=7
  LoaScaDi : Inport  RequirementInfo={} %GIDa_222cbc6c_4673_425c_9331_7d48f6fb500b  Port=8
  function : TriggerPort  TriggerType=function-call
  Arbitrate_Responses : Subsystem
  Assign_Scale : Subsystem
  Calc_Ivtr_State : Subsystem
  Demux : Demux
  If : If  RequirementInfo="{'linktype_rmi_doors' '00012fd5 (/E-STEER Core/SubSystem Specifications/Application Functions - EA4/SF049A Loss of Assist Manager)' '#SF049A_104' 'true' 'REQ:  SF049A_104' '' } %GIDa_f10a060e_1707_4b4d_a14f_31f60975eb58"  IfExpression=u1
  Latch_Inputs : Subsystem
  LimLoa : NxtrLim/LimStat_f32  RequirementInfo={} %GIDa_a349ea4d_a856_44b5_bab4_132edc606aaf  LoLim=LOASCAZERO_ULS_F32  HiLim=LOASCAONE_ULS_F32
      settings: AttributesFormatString=|
      | Low Limit: %<LoLim>
      | High Limit:%<HiLim>
  LimLoaRate : NxtrLim/LimStat_f32  RequirementInfo={} %GIDa_9955eddd_8e62_4c77_871d_df6e2ee160e9  LoLim=LOAMINSLEW_ULSPERSEC_F32  HiLim=LOAMAXSLEW_ULSPERSEC_F32
      settings: AttributesFormatString=|
      | Low Limit: %<LoLim>
      | High Limit:%<HiLim>
  Merge : Merge  RequirementInfo="{'linktype_rmi_doors' '00012fd5 (/E-STEER Core/SubSystem Specifications/Application Functions - EA4/SF049A Loss of Assist Manager)' '#SF049A_104' 'true' 'REQ:  SF049A_104' '' } %GIDa_327415ad_8ba4_4a4e_a51c_70892357edf8"
  Mux : Mux
  Request_Responses : Subsystem
  Set_Faults : Subsystem
  else : Subsystem  RequirementInfo="{'linktype_rmi_doors' '00012fd5 (/E-STEER Core/SubSystem Specifications/Application Functions - EA4/SF049A Loss of Assist Manager)' '#SF049A_104' 'true' 'REQ:  SF049A_104' '' } %GIDa_5728ba8b_03fd_4512_8876_3b4a8063a78e"  TreatAsAtomicUnit=on
  if : Subsystem  RequirementInfo="{'linktype_rmi_doors' '00012fd5 (/E-STEER Core/SubSystem Specifications/Application Functions - EA4/SF049A Loss of Assist Manager)' '#SF049A_104' 'true' 'REQ:  SF049A_104' '' } %GIDa_be9401b4_2311_44f0_8b97_7ac382c4d950"  TreatAsAtomicUnit=on
  LoaSt : Outport
  LoaSca : Outport  Port=2
  LoaRateLim : Outport  Port=3
  HwTqLoaMtgtnEna : Outport  RequirementInfo={} %GIDa_de8377f6_5405_4e42_9e44_71555e1d8f64  Port=4
  MotAgLoaMtgtnEna : Outport  RequirementInfo={} %GIDa_2bcad279_5cb8_4044_9c80_8204913ca898  Port=5
  CurrMeasLoaMtgtnEna : Outport  RequirementInfo={} %GIDa_7b8012c2_a285_40d2_90e0_c53ee278c543  Port=6
  IvtrLoaMtgtnEna : Outport  RequirementInfo={} %GIDa_ac26e2d1_9e7b_47e4_affc_90066996fecc  Port=7
  wires:
  [LoaScaDi] -> If/1
  Assign_Scale/1(LoaSca) -> else/1(In1)
  Merge/1 -> LimLoa/1
  else/1(Out1) -> Merge/2
  if/1(Out1) -> Merge/1
  If/2 -> else/Action
  If/1 -> if/Action
  LimLoa/1 -> LoaSca/1
  LoaScaDi/1 -> [LoaScaDi]
  LimLoaRate/1 -> LoaRateLim/1
  Assign_Scale/2(LoaRate) -> LimLoaRate/1
  Demux/4 -> IvtrLoaMtgtnEna/1
  Demux/2 -> MotAgLoaMtgtnEna/1
  Demux/3 -> CurrMeasLoaMtgtnEna/1
  Demux/1 -> HwTqLoaMtgtnEna/1
  Arbitrate_Responses/2(SwMtgtnEnMux) -> Assign_Scale/2(SwMtgtnEnMux), Demux/1
  Arbitrate_Responses/1(LoaState) -> Assign_Scale/1(LoaSt), LoaSt/1, Set_Faults/2(LoaState)
  Request_Responses/1(RespMux) -> Arbitrate_Responses/1(RespMux)
  MotAgSnsrlsAvl/1 -> Request_Responses/3(MotAgSnsrlsAvl)
  TqLoaAvl/1 -> Request_Responses/2(TqLoaAvl)
  Latch_Inputs/1(SigCntMux) -> Request_Responses/1(SigCntMux), Set_Faults/1(SignalCountMux)
  MotAgMeclIdptSig/1 -> Mux/2
  DiagcStsIvtr2Inactv/1 -> Calc_Ivtr_State/2(Ivtr2Inactv)
  DiagcStsIvtr1Inactv/1 -> Calc_Ivtr_State/1(Ivtr1Inactv)
  CurrMeasIdptSig/1 -> Mux/3
  Calc_Ivtr_State/1(IvtrIdptSig) -> Mux/4  "IvtrIdptSig"
  Mux/1 -> Latch_Inputs/1(RawSigCntMux)
  HwTqIdptSig/1 -> Mux/1

== system SF049A_LoaMgr/call_LoaMgrInit1/CopyRight2 ==

== system SF049A_LoaMgr/call_LoaMgrPer1/CopyRight2 ==

== system SF049A_LoaMgr/ISO Fault Debounce/DiagMgr/CopyRight2 ==

== system SF049A_LoaMgr/ISO Fault Debounce/DiagMgr/If Action Subsystem ==
  EA : Inport
  Qlf : Inport  Port=2
  Action Port : ActionPort  ActionType=else
  EAo : Outport
  Qlfo : Outport  Port=2
  wires:
  EA/1 -> EAo/1
  Qlf/1 -> Qlfo/1

== system SF049A_LoaMgr/ISO Fault Debounce/DiagMgr/If Action Subsystem1 ==
  Qlf : Inport
  EA : Inport  Port=2
  Action Port : ActionPort  ActionType=then
  Qlfo : Outport
  EAo : Outport  Port=2
  wires:
  EA/1 -> EAo/1
  Qlf/1 -> Qlfo/1

== system SF049A_LoaMgr/ISO Fault Debounce/DiagMgr/If Action Subsystem3 ==
  In1 : Inport
  Action Port : ActionPort  ActionType=then
  Out1 : Outport
  wires:
  In1/1 -> Out1/1

== system SF049A_LoaMgr/ISO Fault Debounce/DiagMgr/If Action Subsystem4 ==
  In1 : Inport
  Action Port : ActionPort  ActionType=else
  Out1 : Outport
  wires:
  In1/1 -> Out1/1

== system SF049A_LoaMgr/ISO Fault Debounce/DiagMgr/NTCSTS_FAILD ==
  EA : Inport
  Qlf : Inport  Port=2
  Action Port : ActionPort  ActionType=case
  EAo : Outport
  Qlfo : Outport  Port=2
  wires:
  EA/1 -> EAo/1
  Qlf/1 -> Qlfo/1

== system SF049A_LoaMgr/ISO Fault Debounce/DiagMgr/NTCSTS_PASSD ==
  EA : Inport
  Qlf : Inport  Port=2
  Action Port : ActionPort  ActionType=case
  EAo : Outport
  Qlfo : Outport  Port=2
  wires:
  EA/1 -> EAo/1
  Qlf/1 -> Qlfo/1
